simulink model "ROSReady_FollowerStopper_v1"  (R2019a)
settings: Solver=FixedStepAuto  StartTime=0.0  StopTime=inf  FixedStep=0.01  RelTol=1e-3
values from neighbouring files (symbols this model uses):
  delta = 1.508    [maxSafeSpeed.m]
libraries: robotlib x10
settings Model: Creator=ckreienk  LastModifiedBy=ivory
settings DataIOCC: ReturnWorkspaceOutputs=off
settings OptimizationCC: EnhancedBackFolding=on  PassReuseOutputArgsAs=Individual arguments  MaxStackSize=64  OptimizeBlockOrder=speed  DifferentSizesBufferReuse=on  OptimizationCustomize=off
settings DebuggingCC: ParameterTunabilityLossMsg=error  ArithmeticOperatorsInVariantConditions=warning
settings HardwareCC: ProdBitPerPointer=32  ProdBitPerSizeT=32  ProdBitPerPtrDiffT=32  ProdLargestAtomicFloat=None  ProdIntDivRoundTo=Undefined  ProdEndianess=Unspecified  ProdWordSize=32  ProdHWDeviceType=Generic->Unspecified (assume 32-bit Generic)
settings SFSimCC: MATLABDynamicMemAlloc=off
settings RTWCC: SystemTargetFile=ert.tlc  HardwareBoard=Robot Operating System (ROS)  TLCOptions="-aInlineSetEventsForThisBaseRateFcn=TLC_FALSE -aSuppressMultiTaskScheduler=TLC_FALSE  -aRateBasedStepFcn=0"  TemplateMakefile=ert_default_tmf  GenerateReport=on  Toolchain=Catkin  IncludeHyperlinkInReport=on  LaunchReport=on  TargetLang=C++  GenerateTraceInfo=on  GenerateTraceReport=on  GenerateTraceReportSl=on  GenerateTraceReportSf=on  GenerateTraceReportEml=on
settings CodeAppCC: ForceParamTrailComments=on  IgnoreCustomStorageClasses=off  OperatorAnnotations=on  SimulinkDataObjDesc=on  SFDataObjDesc=on  InsertBlockDesc=on
settings ERTTargetCC: SupportVariableSizeSignals=on

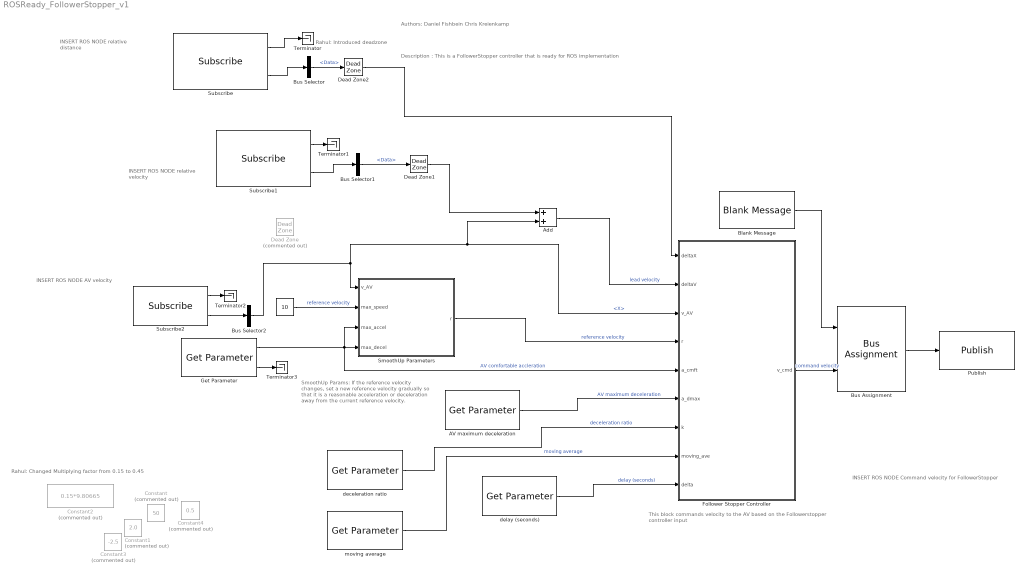
== system ROSReady_FollowerStopper_v1 ==
  note: Rahul: Changed Multiplying factor from 0.15 to 0.45
  note: Description : This is a FollowerStopper controller that is ready for ROS implementation
  note: Authors: Daniel Fishbein
      | Chris Kreienkamp
  note: INSERT ROS NODE
      | relative velocity
  note: INSERT ROS NODE
      | AV velocity
  note: INSERT ROS NODE
      | Command velocity for FollowerStopper
  note: SmoothUp Params:
      | If the reference velocity changes,
      | set a new reference velocity gradually
      | so that it is a reasonable acceleration
      | or deceleration away from the current
      | reference velocity.
  note: This block commands velocity to the AV based
      | on the Followerstopper controller input
  note: INSERT ROS NODE
      | relative distance
  note: Rahul: Introduced deadzone
  " " : Constant  Value=10
  AV maximum deceleration : robotlib/Get Parameter  ParameterSource=Specify your own  ParameterName=/decel_max  ParameterType=double  ParameterMaxArrayLength=16  ParameterInitialValue=-2.50  SampleTime=-1  ShowErrorCodeOutput=off  ModelName=ROSReady_FollowerStopper_v1  BlockId=ParamGet_ROSReady_FollowerStopper_v1_1389
      settings: SourceProductName=Robotics System Toolbox  SourceProductBaseCode=RO
  Add : Sum
  Blank Message : robotlib/Blank Message  messageClass=Message  entityType=geometry_msgs/Twist  messageType=geometry_msgs/Twist  SampleTime=inf
      settings: SourceProductBaseCode=RO
  Bus Assignment : BusAssignment  AssignedSignals=Linear.X
  Bus Selector : BusSelector  OutputSignals=Data
  Bus Selector1 : BusSelector  OutputSignals=Data
  Bus Selector2 : BusSelector  OutputSignals=Linear.X
  Constant : Constant  Commented=on  Value=50
  Constant1 : Constant  Commented=on  Value=2.0
  Constant2 : Constant  Commented=on  Value=0.15*9.80665
  Constant3 : Constant  Commented=on  Value=-2.5
  Constant4 : Constant  Commented=on  Value=0.5
  Dead Zone : DeadZone  Commented=on  LowerValue=-0.1  UpperValue=0.1  SaturateOnIntegerOverflow=on
  Dead Zone1 : DeadZone  LowerValue=-0.1  UpperValue=0.1  SaturateOnIntegerOverflow=on
  Dead Zone2 : DeadZone  LowerValue=-0.1  UpperValue=0.1  SaturateOnIntegerOverflow=on
  Follower Stopper Controller : Subsystem
  Get Parameter : robotlib/Get Parameter  ParameterSource=Specify your own  ParameterName=/accel_cm  ParameterType=double  ParameterMaxArrayLength=16  ParameterInitialValue=0.15*9.80665  SampleTime=-1  ShowErrorCodeOutput=on  ModelName=ROSReady_FollowerStopper_v1  BlockId=ParamGet_ROSReady_FollowerStopper_v1_1385
      settings: SourceProductName=Robotics System Toolbox  SourceProductBaseCode=RO
  Publish : robotlib/Publish  topicSource=Specify your own  topic=cmd_vel  messageType=geometry_msgs/Twist  messageQueueLength=1
      settings: SourceProductBaseCode=RO
  SmoothUp Parameters : MATLAB Function  TreatAsAtomicUnit=on
  Subscribe : robotlib/Subscribe  topicSource=Specify your own  topic=relativeDistance  messageType=std_msgs/Float64  sampleTime=-1  messageQueueLength=1
      settings: SourceProductBaseCode=RO
  Subscribe1 : robotlib/Subscribe  topicSource=Specify your own  topic=relativeVel  messageType=std_msgs/Float64  sampleTime=-1  messageQueueLength=1
      settings: SourceProductBaseCode=RO
  Subscribe2 : robotlib/Subscribe  topicSource=Specify your own  topic=vel  messageType=geometry_msgs/Twist  sampleTime=-1  messageQueueLength=1
      settings: SourceProductBaseCode=RO
  Terminator{,1..3} (4 alike) : Terminator
  deceleration ratio : robotlib/Get Parameter  ParameterSource=Specify your own  ParameterName=/decel_ratio  ParameterType=double  ParameterMaxArrayLength=16  ParameterInitialValue=2.0  SampleTime=-1  ShowErrorCodeOutput=off  ModelName=ROSReady_FollowerStopper_v1  BlockId=ParamGet_ROSReady_FollowerStopper_v1_1391
      settings: SourceProductName=Robotics System Toolbox  SourceProductBaseCode=RO
  delay (seconds) : robotlib/Get Parameter  ParameterSource=Specify your own  ParameterName=/delta  ParameterType=double  ParameterMaxArrayLength=16  ParameterInitialValue=0.5  SampleTime=-1  ShowErrorCodeOutput=off  ModelName=ROSReady_FollowerStopper_v1  BlockId=ParamGet_ROSReady_FollowerStopper_v1_1395
      settings: SourceProductName=Robotics System Toolbox  SourceProductBaseCode=RO
  moving average : robotlib/Get Parameter  ParameterSource=Specify your own  ParameterName=/moving_avg  ParameterType=int32  ParameterMaxArrayLength=16  ParameterInitialValue=50  SampleTime=-1  ShowErrorCodeOutput=off  ModelName=ROSReady_FollowerStopper_v1  BlockId=ParamGet_ROSReady_FollowerStopper_v1_1393
      settings: SourceProductName=Robotics System Toolbox  SourceProductBaseCode=RO
  wires:
  SmoothUp Parameters/1(r) -> Follower Stopper Controller/4(r)  "reference velocity"
  moving average/1 -> Follower Stopper Controller/8(moving_ave)  "moving average"
  Follower Stopper Controller/1(v_cmd) -> Bus Assignment/2  "command velocity"
  AV maximum deceleration/1 -> Follower Stopper Controller/6(a_dmax)  "AV maximum deceleration"
  " "/1 -> SmoothUp Parameters/2(max_speed)  "reference velocity"
  deceleration ratio/1 -> Follower Stopper Controller/7(k)  "deceleration ratio"
  Add/1 -> Follower Stopper Controller/2(deltaV)  "lead velocity"
  Bus Selector/1 -> Dead Zone2/1  "<Data>"
  Get Parameter/1 -> Follower Stopper Controller/5(a_cmft), SmoothUp Parameters/3(max_accel), SmoothUp Parameters/4(max_decel)  "AV comfortable accleration"
  Bus Selector2/1 -> Add/2, Follower Stopper Controller/3(v_AV), SmoothUp Parameters/1(v_AV)  "<X>"
  Bus Selector1/1 -> Dead Zone1/1  "<Data>"
  delay (seconds)/1 -> Follower Stopper Controller/9(delta)  "delay (seconds)"
  Subscribe/2 -> Bus Selector/1
  Subscribe/1 -> Terminator/1
  Subscribe1/1 -> Terminator1/1
  Subscribe1/2 -> Bus Selector1/1
  Subscribe2/1 -> Terminator2/1
  Subscribe2/2 -> Bus Selector2/1
  Blank Message/1 -> Bus Assignment/1
  Bus Assignment/1 -> Publish/1
  Dead Zone1/1 -> Add/1
  Dead Zone2/1 -> Follower Stopper Controller/1(deltaX)
  Get Parameter/2 -> Terminator3/1

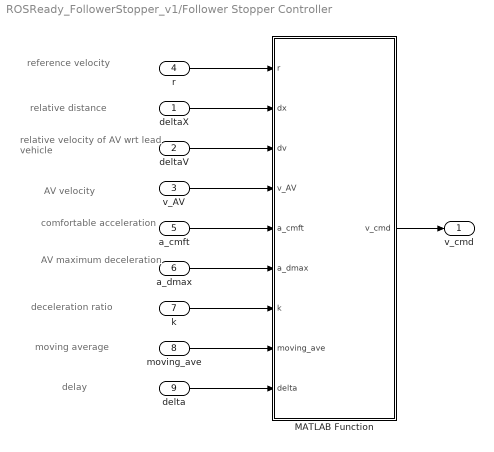
== system ROSReady_FollowerStopper_v1/Follower Stopper Controller ==
  note: relative distance
  note: reference velocity
  note: AV velocity
  note: relative velocity of
      | AV wrt lead vehicle
  note: comfortable
      | acceleration
  note: AV maximum
      | deceleration
  note: deceleration ratio
  note: moving average
  note: delay
  deltaX : Inport
  deltaV : Inport  Port=2
  v_AV : Inport  Port=3
  r : Inport  Port=4
  a_cmft : Inport  Port=5
  a_dmax : Inport  Port=6
  k : Inport  Port=7
  moving_ave : Inport  Port=8
  delta : Inport  Port=9
  MATLAB Function : MATLAB Function  TreatAsAtomicUnit=on
  v_cmd : Outport
  wires:
  r/1 -> MATLAB Function/1(r)
  v_AV/1 -> MATLAB Function/4(v_AV)
  MATLAB Function/1(v_cmd) -> v_cmd/1
  deltaV/1 -> MATLAB Function/3(dv)
  deltaX/1 -> MATLAB Function/2(dx)
  moving_ave/1 -> MATLAB Function/8(moving_ave)
  a_cmft/1 -> MATLAB Function/5(a_cmft)
  a_dmax/1 -> MATLAB Function/6(a_dmax)
  k/1 -> MATLAB Function/7(k)
  delta/1 -> MATLAB Function/9(delta)

== matlab function ROSReady_FollowerStopper_v1/Follower Stopper Controller/MATLAB Function ==
  settings: updateMethod=DISCRETE
  data: r input; dx input; dv input; v_cmd output; v_AV input; a_cmft input; a_dmax input; k input; moving_ave input; delta input
function v_cmd = fcn(r,dx,dv,v_AV,...
    a_cmft, a_dmax, k, moving_ave, delta)

%#codegen
% Safety controller, based on quadratic bands.
% Input: r = desired velocity (from other models)
%          dx = estimate of gap to vehicle ahead
%          dv = estimate of time derivative of dx (= velocity difference)
%        v_AV = velocity of AV
%      a_cmft = comfortable acceleration
%      a_dmax = maximum AV deceleration
%           k = ratio between maximum lead deceleration and a_dmax
%  moving_ave = number of v_cmd data points of which to take the average
% Out:  v_cmd = actual velocity commanded (always v_cmd<=r)
%
% Controller-specific parameters

% Lead vehicle velocity
v_lead = v_AV+dv; % velocity of lead vehicle
v_lead = max(v_lead,0); % lead vehicle cannot go backwards
v = min(r,v_lead); % safety velocity cannot exceed desired velocity r

% Relative distance parameters
deltaVSStar = max(1/(2*k*a_dmax)*(v_lead^2-k*v_AV^2),0);
dx1 = 1+deltaVSStar+v_AV*(1-a_cmft/a_dmax)*delta+a_cmft/2*(1-a_cmft/a_dmax)*delta^2;
dx2 = dx1 + 2*v_AV*delta;
dx3 = 2*dx2-dx1;

% Actual commanded velocity
dt = 0.01;
smoothChange = v_AV + a_cmft*dt;
new_cmd = double((dx<=dx1).*(0))+...
    (dx1<dx&dx<=dx2).*(min(v*(dx-dx1)/(dx2-dx1) , smoothChange))+...
    (dx2<dx&dx<=dx3).*(min(v + (r-v)*(dx-dx2)/(dx3-dx2) , smoothChange))+...
    (dx3<dx).*(min(r , smoothChange));

% Take moving average of last moving_ave number of values
persistent moving_array
if isempty(moving_array)
    moving_array=zeros(1,int8(moving_ave));
end
moving_array = [moving_array(2:int8(moving_ave)) new_cmd];

% Use the maximum of the moving average and the AV velocity achieved if
% maximum braking is used
fastestDecel = v_AV + a_dmax*dt;
v_cmd = max(mean(moving_array,'all'),fastestDecel);

== matlab function ROSReady_FollowerStopper_v1/SmoothUp Parameters ==
  settings: updateMethod=DISCRETE
  data: v_AV input; max_speed input; r output; max_accel input; max_decel input
function r = fcn(v_AV,max_speed,max_accel,max_decel)
% #codegen
persistent y

if isempty(y)
    y=v_AV;
end

dt=0.01;
if( y > max_speed + max_accel*dt)
    y = max(max_speed,y - abs(max_decel)*dt);
elseif( y < max_speed - abs(max_decel)*dt)
    y = min(max_speed,y + max_accel*dt);
else
    y = max_speed;
end

r = y;
